simulink model "lecture09d_model"  (R2021a)
settings: Solver=ode3  StartTime=0.0  StopTime=t_final  FixedStep=t_sample  MaxStep=.05  RelTol=1e-3  EnableMultiTasking=on
values from neighbouring files (symbols this model uses):
  A = temp.A    [lecture09d.m]    (also in linear_model_straight_level.mat = [-0.035373280601 0 -0.219927945485 0 -0.00100878120672 0 0 0)
  B = temp.B    [lecture09d.m]    (also in linear_model_straight_level.mat = [0 0 0 -0.948606836678 0 -0.0198636151401 0 0 0 0.1094304025)
  C = temp.C    [lecture09d.m]    (also in linear_model_straight_level.mat = [1 0 0 0 0 0 0 0 0 0 1 0 ... (81 elements, 9x9)])
  D = temp.D    [lecture09d.m]    (also in linear_model_straight_level.mat = [0 0 0 0 0 0 0 0 0 0 0 0 ... (45 elements, 9x5)])
  Delta_x0 = [ ... (first row only)    [lecture09d.m]
  doublet_duration = 5    [lecture09d.m]
  doublet_mag = 0*pi/180    (= 0)    [lecture09d.m]
  uo = temp.UStar    [lecture09d.m]
  xo = temp.XStar    [lecture09d.m]
  yo = xo    [lecture09d.m]
undefined symbols (not defined in the file or in its folder): RCAM_model
settings Model: Creator=lum  LastModifiedBy=chris
settings SolverCC: AlgebraicLoopSolver=TrustRegion
settings DataIOCC: LimitDataPoints=on  SaveFormat=Array  SignalLoggingSaveFormat=ModelDataLogs  ReturnWorkspaceOutputs=off  SignalLoggingName=sigsOut
settings OptimizationCC: ExpressionDepthLimit=2147483647  InitFltsAndDblsToZero=on  LifeSpan=inf
settings DebuggingCC: SaveWithParameterizedLinksMsg=none  UnderspecifiedInitializationDetection=Classic  MergeDetectMultiDrivingBlocksExec=none  SignalResolutionControl=TryResolveAllWithWarning  MultiTaskDSMMsg=warning  MultiTaskCondExecSysMsg=none  FcnCallInpInsideContextMsg=warning  StateNameClashWarn=warning  SFUnexpectedBacktrackingDiag=warning  SFNoUnconditionalDefaultTransitionDiag=warning  SFExecutionAtInitializationDiag=none  SFMachineParentedDataDiag=warning  ArithmeticOperatorsInVariantConditions=warning
settings HardwareCC: ProdBitPerPointer=32  ProdBitPerSizeT=32  ProdBitPerPtrDiffT=32  ProdLargestAtomicFloat=None  ProdIntDivRoundTo=Undefined  ProdEndianess=Unspecified  ProdWordSize=32  ProdHWDeviceType=32-bit Generic  TargetUnknown=on
settings ModelReferenceCC: PropagateSignalLabelsOutOfModel=off
settings SFSimCC: SimParseCustomCode=off  CustomCodeUndefinedFunction=UseInterfaceOnly
settings CodeAppCC: StateflowObjectComments=on
settings GRTTargetCC: TargetFcnLib=ansi_tfl_tmw.mat  TargetLangStandard=C89/C90 (ANSI)  ModelReferenceCompliant=off  CombineOutputUpdateFcns=off  MatFileLogging=off  GRTInterface=on
settings ConfigComp: CovMetricSettings=dw  CovSaveCumulativeToWorkspaceVar=on  CovSaveSingleToWorkspaceVar=on

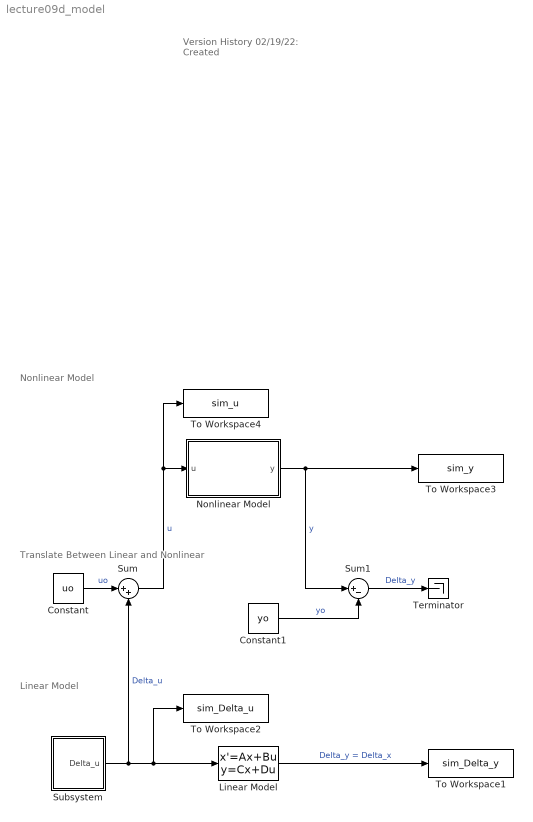
== system lecture09d_model ==
  note: Translate Between Linear and Nonlinear
  note: Linear Model
  note: Nonlinear Model
  note: Version History
      | 02/19/22: Created
  Constant : Constant  Value=uo
  Constant1 : Constant  Value=yo
  Linear Model : StateSpace  A=A  B=B  C=C  D=D  InitialCondition=Delta_x0
  "Nonlinear Model " : Subsystem
  Subsystem : Subsystem
  Sum : Sum  Inputs=|++
  Sum1 : Sum  Inputs=|+-
  Terminator : Terminator
  To Workspace1 : ToWorkspace  VariableName=sim_Delta_y  SaveFormat=Structure With Time  SampleTime=-1
  To Workspace2 : ToWorkspace  VariableName=sim_Delta_u  SaveFormat=Structure With Time  SampleTime=-1
  To Workspace3 : ToWorkspace  VariableName=sim_y  SaveFormat=Structure With Time  SampleTime=-1
  To Workspace4 : ToWorkspace  VariableName=sim_u  SaveFormat=Structure With Time  SampleTime=-1
  wires:
  Constant/1 -> Sum/1  "uo"
  "Nonlinear Model "/1(y) -> To Workspace3/1, Sum1/1  "y"
  Subsystem/1(Delta_u) -> To Workspace2/1, Linear Model/1, Sum/2  "Delta_u"
  Linear Model/1 -> To Workspace1/1  "Delta_y = Delta_x"
  Sum/1 -> To Workspace4/1, "Nonlinear Model "/1(u)  "u"
  Constant1/1 -> Sum1/2  "yo"
  Sum1/1 -> Terminator/1  "Delta_y"

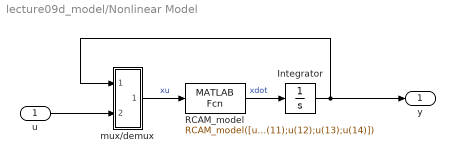
== system lecture09d_model/Nonlinear Model  ==
  u : Inport
  Integrator : Integrator  InitialCondition=xo+Delta_x0
  RCAM_model : MATLABFcn  MATLABFcn=RCAM_model([u(1);u(2);u(3);u(4);u(5);u(6);u(7);u(8);u(9)],[u(10);u(11);u(12);u(13);u(14)])
  mux/demux : Subsystem
  y : Outport  VectorParamsAs1DForOutWhenUnconnected=off
  wires:
  u/1 -> mux/demux/2(u)
  RCAM_model/1 -> Integrator/1  "xdot"
  mux/demux/1(xu) -> RCAM_model/1  "xu"
  Integrator/1 -> y/1, mux/demux/1(x)

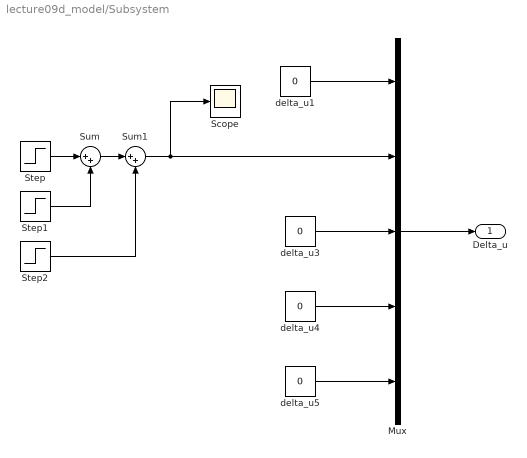
== system lecture09d_model/Subsystem ==
  Mux : Mux  Inputs=5
  Scope : Scope
  Step : Step  Time=5  After=doublet_mag  SampleTime=0
  Step1 : Step  Time=5+doublet_duration  After=-2*doublet_mag  SampleTime=0
  Step2 : Step  Time=5+2*doublet_duration  After=doublet_mag  SampleTime=0
  Sum : Sum  Inputs=|++  SaturateOnIntegerOverflow=on
  Sum1 : Sum  Inputs=|++  SaturateOnIntegerOverflow=on
  delta_u{1,3..5} (4 alike) : Constant  Value=0
  Delta_u : Outport  VectorParamsAs1DForOutWhenUnconnected=off
  wires:
  delta_u5/1 -> Mux/5
  delta_u4/1 -> Mux/4
  delta_u3/1 -> Mux/3
  delta_u1/1 -> Mux/1
  Mux/1 -> Delta_u/1
  Sum1/1 -> Scope/1, Mux/2
  Step2/1 -> Sum1/2
  Sum/1 -> Sum1/1
  Step1/1 -> Sum/2
  Step/1 -> Sum/1

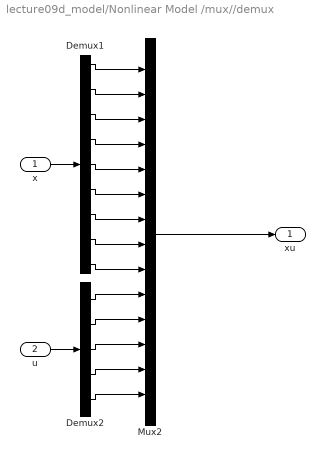
== system lecture09d_model/Nonlinear Model /mux//demux ==
  x : Inport
  u : Inport  Port=2
  Demux1 : Demux  Outputs=9
      settings: DisplayOption=none
  Demux2 : Demux  Outputs=5
      settings: DisplayOption=none
  Mux2 : Mux  Inputs=14
  xu : Outport  VectorParamsAs1DForOutWhenUnconnected=off
  wires:
  Demux2/5 -> Mux2/14
  Demux2/4 -> Mux2/13
  Demux2/3 -> Mux2/12
  Demux2/2 -> Mux2/11
  Demux2/1 -> Mux2/10
  Demux1/9 -> Mux2/9
  Demux1/8 -> Mux2/8
  Demux1/7 -> Mux2/7
  Demux1/6 -> Mux2/6
  Demux1/5 -> Mux2/5
  Demux1/4 -> Mux2/4
  Demux1/3 -> Mux2/3
  Demux1/2 -> Mux2/2
  Demux1/1 -> Mux2/1
  u/1 -> Demux2/1
  Mux2/1 -> xu/1
  x/1 -> Demux1/1
